simulink model "droop_model_with_current_limitation"  (R2018a)
settings: Solver=ode23tb  StartTime=0.0  StopTime=Tend  RelTol=1e-3
values from neighbouring files (symbols this model uses):
  C_4 = 0.1670*C_b    (= 1.00487241952e-06)    [VSM.m]    (also in dVOC.m; droop.m; droop_with_current_limitation.m; matching.m)
  C_6 = 0.2835*C_b    (= 1.70587623314e-06)    [VSM.m]    (also in dVOC.m; droop.m; droop_with_current_limitation.m; matching.m)
  C_8 = 0.2275*C_b    (= 1.36891302659e-06)    [VSM.m]    (also in dVOC.m; droop.m; droop_with_current_limitation.m; matching.m)
  C_dc = 0.008*(n)    (= 1.6)    [VSM.m]    (also in dVOC.m; droop.m; droop_with_current_limitation.m; matching.m)
  C_f = n*300*10^-6    (= 0.06)    [VSM.m]    (also in dVOC.m; droop.m; droop_with_current_limitation.m; matching.m)
  droop_percentage = 1    [VSM.m]    (also in dVOC.m; droop.m; droop_with_current_limitation.m; matching.m)
  I_b_LV = S_b/(sqrt(3)*V1_rms)    [VSM.m]    (also in dVOC.m; droop.m; droop_with_current_limitation.m = sqrt(2)*S_b/(sqrt(3)*V1_rms); matching.m)
  i_ll = -1.15*(S_b/Vdc_n)-i_loss_dc    [VSM.m]    (also in dVOC.m; droop.m; droop_with_current_limitation.m; matching.m)
  i_ul = 1.15*(S_b/Vdc_n)+i_loss_dc    [VSM.m]    (also in dVOC.m; droop.m; droop_with_current_limitation.m; matching.m)
  idppu = 0.9    [droop_with_current_limitation.m]
  isatpu = 1.2    [droop_with_current_limitation.m]
  k_dc = eta_1/(Vdc_n*m_p)    [VSM.m]    (also in dVOC.m; droop.m; droop_with_current_limitation.m; matching.m)
  K_dP = 2.3*S_b    (= 230000000)    [droop_with_current_limitation.m]
  K_p = (1/Vdc_n)    [VSM.m]    (also in dVOC.m; droop.m; droop_with_current_limitation.m; matching.m)
  K_r = 1/R_dc    [VSM.m]    (also in dVOC.m; droop.m; droop_with_current_limitation.m; matching.m)
  Kff_i = 1    [VSM.m]    (also in dVOC.m; droop.m; droop_with_current_limitation.m; matching.m)
  Kff_v = 1    [VSM.m]    (also in dVOC.m; droop.m; droop_with_current_limitation.m; matching.m)
  Ki_i = (1/n)*1.19    (= 0.00595)    [VSM.m]    (also in dVOC.m; droop.m; droop_with_current_limitation.m; matching.m)
  Ki_v = (n)*1.161022    (= 232.2044)    [VSM.m]    (also in dVOC.m; droop.m; droop_with_current_limitation.m; matching.m)
  ki_v_ac = 4*5.2500e-04    (= 0.0021)    [VSM.m]    (also in dVOC.m = 0.5; droop.m = 0.5; droop_with_current_limitation.m = 0.5; matching.m = 0.5)
  Kp_i = 0.738891    [VSM.m]    (also in dVOC.m; droop.m; droop_with_current_limitation.m; matching.m)
  Kp_v = 0.52    [VSM.m]    (also in dVOC.m; droop.m; droop_with_current_limitation.m; matching.m)
  kp_v_ac = 0.001    [VSM.m]    (also in dVOC.m; droop.m; droop_with_current_limitation.m; matching.m)
  L1_pu = 1*0.0186/m    (= 0.000186)    [VSM.m]    (also in dVOC.m; droop.m; droop_with_current_limitation.m; matching.m)
  L_45 = L_lines(2)    [VSM.m]    (also in dVOC.m; droop.m; droop_with_current_limitation.m; matching.m)
  L_56 = L_lines(3)    [VSM.m]    (also in dVOC.m; droop.m; droop_with_current_limitation.m; matching.m)
  L_67 = L_lines(5)    [VSM.m]    (also in dVOC.m; droop.m; droop_with_current_limitation.m; matching.m)
  L_78 = L_lines(6)    [VSM.m]    (also in dVOC.m; droop.m; droop_with_current_limitation.m; matching.m)
  L_89 = L_lines(8)    [VSM.m]    (also in dVOC.m; droop.m; droop_with_current_limitation.m; matching.m)
  L_94 = L_lines(9)    [VSM.m]    (also in dVOC.m; droop.m; droop_with_current_limitation.m; matching.m)
  L_f = (1/n)*200*10^-6    (= 1e-06)    [VSM.m]    (also in dVOC.m; droop.m; droop_with_current_limitation.m; matching.m)
  m_p = (2*pi*0.5)/(S_b)    (= 3.14159265359e-08)    [VSM.m]    (also in dVOC.m; droop.m; droop_with_current_limitation.m; matching.m)
  n = 200    [VSM.m]    (also in dVOC.m; droop.m; droop_with_current_limitation.m; matching.m)
  ps = base/3    (= 0.75)    [VSM.m]    (also in dVOC.m; droop.m; droop_with_current_limitation.m; matching.m)
  R1_pu = 1*0.00734/m    (= 7.34e-05)    [VSM.m]    (also in dVOC.m; droop.m; droop_with_current_limitation.m; matching.m)
  R_45 = R_lines(2)    [VSM.m]    (also in dVOC.m; droop.m; droop_with_current_limitation.m; matching.m)
  R_56 = R_lines(3)    [VSM.m]    (also in dVOC.m; droop.m; droop_with_current_limitation.m; matching.m)
  R_67 = R_lines(5)    [VSM.m]    (also in dVOC.m; droop.m; droop_with_current_limitation.m; matching.m)
  R_78 = R_lines(6)    [VSM.m]    (also in dVOC.m; droop.m; droop_with_current_limitation.m; matching.m)
  R_89 = R_lines(8)    [VSM.m]    (also in dVOC.m; droop.m; droop_with_current_limitation.m; matching.m)
  R_94 = R_lines(9)    [VSM.m]    (also in dVOC.m; droop.m; droop_with_current_limitation.m; matching.m)
  R_dc = (Vdc_n/(0.05*(S_b)/Vdc_n))    [VSM.m]    (also in dVOC.m; droop.m; droop_with_current_limitation.m; matching.m)
  R_f = 0.001/n    (= 5e-06)    [VSM.m]    (also in dVOC.m; droop.m; droop_with_current_limitation.m; matching.m)
  S_b = 100*(10^6)    (= 100000000)    [VSM.m]    (also in dVOC.m; droop.m; droop_with_current_limitation.m; matching.m)
  S_bt = S_b    (= 100000000)    [VSM.m]    (also in dVOC.m; droop.m; droop_with_current_limitation.m; matching.m)
  T_en = T_load-0.5    (= 24.5)    [VSM.m]    (also in dVOC.m; droop.m; droop_with_current_limitation.m; matching.m)
  T_load = 25    [VSM.m]    (also in dVOC.m; droop.m; droop_with_current_limitation.m; matching.m)
  T_loss = Tend    (= 50)    [dVOC.m]    (also in droop.m; droop_with_current_limitation.m)
  T_ms = 0.001    [dVOC.m]    (also in droop.m; droop_with_current_limitation.m)
  T_s = 1e-4    (= 0.0001)    [VSM.m]    (also in dVOC.m; droop.m; droop_with_current_limitation.m; matching.m)
  tau_dc = 0.05    [VSM.m]    (also in dVOC.m; droop.m; droop_with_current_limitation.m; matching.m)
  tau_g = 5    [VSM.m]    (also in dVOC.m; droop.m; droop_with_current_limitation.m; matching.m)
  V1_rms = 1000    [VSM.m]    (also in dVOC.m; droop.m; droop_with_current_limitation.m; matching.m)
  V2_rms = 13800    [VSM.m]    (also in dVOC.m; droop.m; droop_with_current_limitation.m; matching.m)
  V_m = sqrt(2/3)*V1_rms    [VSM.m]    (also in dVOC.m; droop.m; droop_with_current_limitation.m; matching.m)
  Vdc_n = 3*V_m    [VSM.m]    (also in dVOC.m; droop.m; droop_with_current_limitation.m; matching.m)
  w_b = 2*pi*f_b    (= 314.159265359)    [VSM.m]    (also in dVOC.m; droop.m; droop_with_current_limitation.m; matching.m)
  w_f = 2*pi*5    (= 31.4159265359)    [VSM.m]    (also in dVOC.m; droop.m; droop_with_current_limitation.m; matching.m)
undefined symbols (not defined in the file or in its folder): D1, Delta, i_dc
libraries: powerlib x88, powerlib_meascontrol x22, cstblocks x3, simulink x2, sps_avr x1
(part 2 of 2)

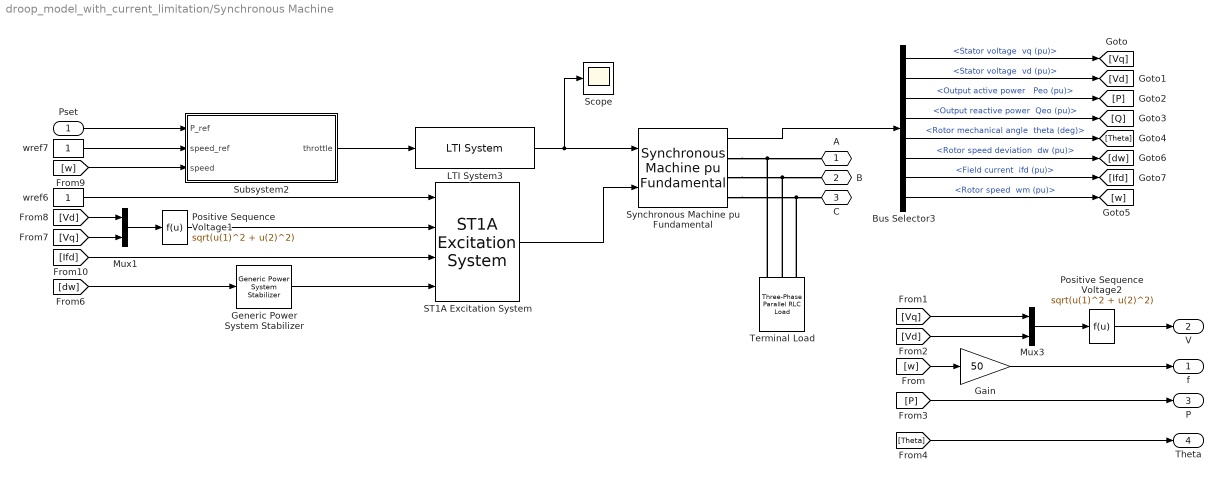
== system droop_model_with_current_limitation/Synchronous Machine ==
  Pset : Inport
  Bus Selector3 : BusSelector  OutputSignals="dq0 components.Stator voltage  vq (pu),dq0 components.Stator voltage  vd (pu),Output active power   Peo (pu),Output reactive power  Qeo (pu),Mechanical.Rotor mechanical angle  theta (deg),Mechanical.Rotor speed deviation  dw (pu),dq0 components.Field current  ifd (pu),Mechanical.Rotor speed  wm (pu)"
  Gain : Gain  Gain=50
  Generic Power System Stabilizer : powerlib/Machines/Generic Power System Stabilizer  Tsensor=30e-4  K=2.5  Twashout=2  Tleadlag1=[2*50e-3 0.1*20e-3]  Tleadlag2=[2*3 0.1*5.4]  VSlimits=2*[-0.15 0.15]  Vinit=0  Plot_On=off  MagdB_On=on  FreqRange=logspace(-2,2,500)
      settings: SourceProductName=Simscape Power Systems  SourceProductBaseCode=PS
  LTI System3 : cstblocks/LTI System  sys=ss(-1/tau_g,1/tau_g,1,[])  IC=ps
  Mux1 : Mux  Inputs=2
  Mux3 : Mux  Inputs=2
  Positive Sequence Voltage1 : Fcn  Expr=sqrt(u(1)^2 + u(2)^2)
  Positive Sequence Voltage2 : Fcn  Expr=sqrt(u(1)^2 + u(2)^2)
  ST1A Excitation System : sps_avr/ST1A Excitation System  Tr=20e-3  KaTa=[210 0.001]  VIminmax=[-999 +999]  VAminmax=[-999 999]  VRminmax=[-6.0 6.43]  KfTf=[0.001 1]  TbTc=[0 0 0 0]  KLR=1  ILR=2  Kc=0.038  v0=[1 1]  TsBlock=0
      settings: SourceProductName=Simscape Power Systems  SourceProductBaseCode=PS
  Scope : Scope
  Subsystem2 : Subsystem
  Synchronous Machine pu Fundamental : powerlib/Machines/Synchronous Machine pu Fundamental  PresetModel=No  MechanicalLoad=Mechanical power Pm  ShowDetailedParameters=on  RotorType=Salient-pole  Units=per unit fundamental parameters  MeasurementBus=off  NominalParameters="[100E6  V2_rms   50]"  Stator="[ 2.85E-03  0.114  1.19  0.36 ]"  Field="[ 5.79E-04  0.114]"  Dampers2=[0.0652, 0.5134, 0.0287, 0.2553, 7.765e-3, 0.9167 ]  Dampers1="[ 1.17E-02  0.182  1.97E-02  0.384 ]"  Mechanical=[ 3.7 0 20]  PolePairs=20  InitialConditions="[ 0  0  0  0  0  0  0  0  1 ]"  SetSaturation=off  Saturation=[0.6404,0.7127,0.8441,0.9214,0.9956,1.082,1.19,1.316,1.457;0.7,0.7698,0.8872,0.9466,0.9969,1.046,1.1,1.151,1.201]  LoadFlowParameters=[1,0,0,0,0]  TsPowergui=0  TsBlock=-1  IterativeModel=Trapezoidal non iterative  IterativeDiscreteModel=Trapezoidal non iterative  BusType=PV  Pref=0  Qref=0  Qmin=-inf  Qmax=inf  PLF=0  QLF=0
      settings: SourceProductName=Simscape Power Systems  SourceProductBaseCode=PS
  Terminal Load : powerlib/Elements/Three-Phase Parallel RLC Load  LConnTagsString=A|B|C  Configuration=Y (grounded)  NominalVoltage=V2_rms  Vabc=[1e3 1e3 1e3]  Vabcp=[1e3 1e3 1e3]  NominalFrequency=50  UnbalancedPower=off  ActivePower=1  InductivePower=0  CapacitivePower=0  Pabc=[10e3 9e3 11e3]  QLabc=[100 90 110]  QCabc=[100 90 110]  Pabcp=[10e3 9e3 11e3]  QLabcp=[100 90 110]  QCabcp=[100 90 110]  Measurements=None  LoadType=constant Z
  wref6 : Constant
  wref7 : Constant
  A : PMIOPort  Side=Right
  B : PMIOPort  Port=2  Side=Right
  C : PMIOPort  Port=3  Side=Right
  f : Outport
  V : Outport  Port=2
  P : Outport  Port=3
  Theta : Outport  Port=4
  wires:
  Gain/1 -> f/1
  Pset/1 -> Subsystem2/1(P_ref)
  Positive Sequence Voltage2/1 -> V/1
  wref7/1 -> Subsystem2/2(speed_ref)
  wref6/1 -> ST1A Excitation System/1
  Mux3/1 -> Positive Sequence Voltage2/1
  Synchronous Machine pu Fundamental/1 -> Bus Selector3/1
  [w] -> Gain/1
  [Vq] -> Mux3/1
  [Vd] -> Mux3/2
  [P] -> P/1
  [Theta] -> Theta/1
  [w] -> Subsystem2/3(speed)
  Subsystem2/1(throttle) -> LTI System3/1
  Bus Selector3/1 -> [Vq]  "<Stator voltage  vq (pu)>"
  Bus Selector3/2 -> [Vd]  "<Stator voltage  vd (pu)>"
  Bus Selector3/3 -> [P]  "<Output active power   Peo (pu)>"
  Bus Selector3/4 -> [Q]  "<Output reactive power  Qeo (pu)>"
  Bus Selector3/5 -> [Theta]  "<Rotor mechanical angle  theta (deg)>"
  Bus Selector3/6 -> [dw]  "<Rotor speed deviation  dw (pu)>"
  Bus Selector3/7 -> [Ifd]  "<Field current  ifd (pu)>"
  Bus Selector3/8 -> [w]  "<Rotor speed  wm (pu)>"
  LTI System3/1 -> Scope/1, Synchronous Machine pu Fundamental/1
  Generic Power System Stabilizer/1 -> ST1A Excitation System/4
  [dw] -> Generic Power System Stabilizer/1
  [Ifd] -> ST1A Excitation System/3
  Mux1/1 -> Positive Sequence Voltage1/1
  [Vd] -> Mux1/1
  [Vq] -> Mux1/2
  Positive Sequence Voltage1/1 -> ST1A Excitation System/2
  ST1A Excitation System/1 -> Synchronous Machine pu Fundamental/2
  connections:
  Terminal Load/LConn1 -- Synchronous Machine pu Fundamental/RConn1 -- A/RConn1
  Terminal Load/LConn3 -- Synchronous Machine pu Fundamental/RConn3 -- C/RConn1
  Terminal Load/LConn2 -- Synchronous Machine pu Fundamental/RConn2 -- B/RConn1

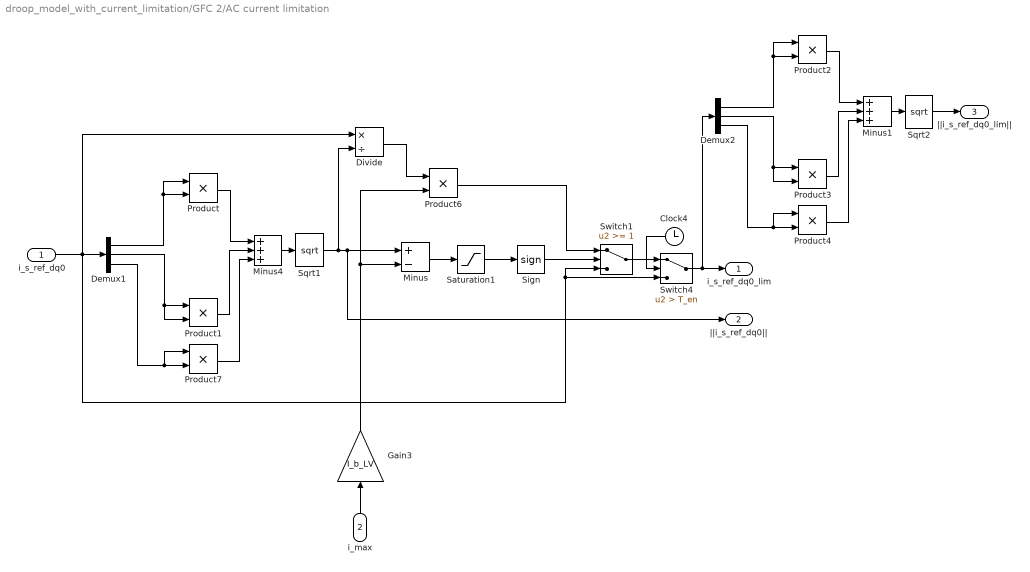
== system droop_model_with_current_limitation/GFC 2/AC current limitation ==
  i_s_ref_dq0 : Inport
  i_max : Inport  Port=2
  Clock4 : Clock
  Demux1 : Demux  Outputs=3
  Demux2 : Demux  Outputs=3
  Divide : Product  Inputs=*/
  Gain3 : Gain  Gain=I_b_LV
  Minus : Sum  Inputs=+-
  Minus1 : Sum  Inputs=+++
  Minus4 : Sum  Inputs=+++
  Product{,1..4,6..7} (7 alike) : Product  RndMeth=Zero
  Saturation1 : Saturate  UpperLimit=inf  LowerLimit=0
  Sign : Signum
  Sqrt1 : Sqrt  SaturateOnIntegerOverflow=on
  Sqrt2 : Sqrt  SaturateOnIntegerOverflow=on
  Switch1 : Switch  Threshold=1
  Switch4 : Switch  Criteria=u2 > Threshold  Threshold=T_en
  i_s_ref_dq0_lim : Outport
  ||i_s_ref_dq0|| : Outport  Port=2
  ||i_s_ref_dq0_lim|| : Outport  Port=3
  wires:
  i_max/1 -> Gain3/1
  Minus/1 -> Saturation1/1
  Sqrt1/1 -> Divide/2, ||i_s_ref_dq0||/1, Minus/1
  Minus4/1 -> Sqrt1/1
  Demux1/1 -> Product/2, Product/1
  Product1/1 -> Minus4/2
  Product/1 -> Minus4/1
  Demux1/2 -> Product1/1, Product1/2
  Saturation1/1 -> Sign/1
  Sign/1 -> Switch1/2
  Divide/1 -> Product6/1
  Product6/1 -> Switch1/1
  Product7/1 -> Minus4/3
  Demux1/3 -> Product7/1, Product7/2
  Switch4/1 -> Demux2/1, i_s_ref_dq0_lim/1
  i_s_ref_dq0/1 -> Divide/1, Demux1/1, Switch4/3, Switch1/3
  Clock4/1 -> Switch4/2
  Switch1/1 -> Switch4/1
  Gain3/1 -> Minus/2, Product6/2
  Product2/1 -> Minus1/1
  Demux2/3 -> Product4/1, Product4/2
  Product4/1 -> Minus1/3
  Demux2/1 -> Product2/2, Product2/1
  Product3/1 -> Minus1/2
  Demux2/2 -> Product3/1, Product3/2
  Minus1/1 -> Sqrt2/1
  Sqrt2/1 -> ||i_s_ref_dq0_lim||/1

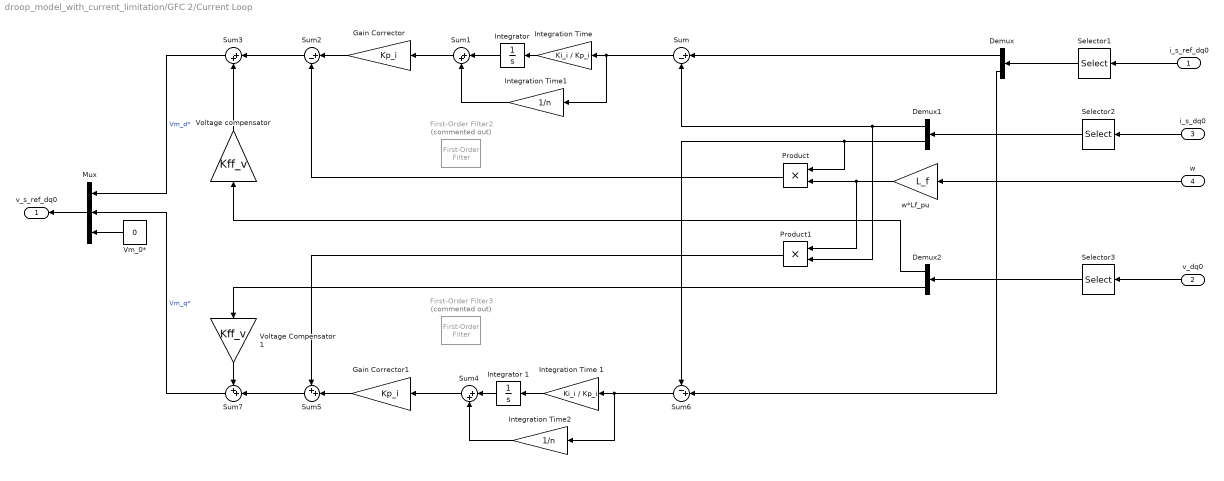
== system droop_model_with_current_limitation/GFC 2/Current Loop ==
  i_s_ref_dq0 : Inport
  v_dq0 : Inport  Port=2
  i_s_dq0 : Inport  Port=3
  w : Inport  Port=4
  Demux : Demux  Outputs=2
  Demux1 : Demux  Outputs=2
  Demux2 : Demux  Outputs=2
  First-Order Filter2 : powerlib_meascontrol/Filters/First-Order Filter  Commented=on  FilterType=Lowpass  Tc=25e-3  Ts=0  Initialize=on  Vac_Init=[0, 0, 50]  Vdc_Init=1  PlotResponse=off  FreqRange="[0,  200,  1]"
      settings: SourceProductName=Simscape Power Systems
  First-Order Filter3 : powerlib_meascontrol/Filters/First-Order Filter  Commented=on  FilterType=Lowpass  Tc=25e-3  Ts=0  Initialize=on  Vac_Init=[0, 0, 50]  Vdc_Init=0  PlotResponse=off  FreqRange="[0,  200,  1]"
      settings: SourceProductName=Simscape Power Systems
  Gain Corrector : Gain  Gain=Kp_i
  Gain Corrector1 : Gain  Gain=Kp_i
  Integration Time : Gain  Gain=Ki_i / Kp_i
  Integration Time 1 : Gain  Gain=Ki_i / Kp_i
  Integration Time1 : Gain  Gain=1/n
  Integration Time2 : Gain  Gain=1/n
  Integrator : Integrator  InitialCondition=0.0001
  Integrator 1 : Integrator
  Mux : Mux  Inputs=3
  Product : Product  RndMeth=Zero
  Product1 : Product  RndMeth=Zero
  Selector1 : Selector  InputPortWidth=3  IndexOptions=Index vector (dialog)  Indices=[1 2]  OutputSizes=1
  Selector2 : Selector  InputPortWidth=3  IndexOptions=Index vector (dialog)  Indices=[1 2]  OutputSizes=1
  Selector3 : Selector  InputPortWidth=3  IndexOptions=Index vector (dialog)  Indices=[1 2]  OutputSizes=1
  Sum : Sum  Inputs=|+-
  Sum1 : Sum  Inputs=|++
  Sum2 : Sum  Inputs=|+-
  Sum3 : Sum  Inputs=|++
  Sum4 : Sum  Inputs=|++
  Sum5 : Sum  Inputs=++|
  Sum6 : Sum  Inputs=-+|
  Sum7 : Sum  Inputs=++|
  Vm_0* : Constant  Value=0
  Voltage Compensator 1 : Gain  Gain=Kff_v
  Voltage compensator : Gain  Gain=Kff_v
  w*Lf_pu : Gain  Gain=L_f
  v_s_ref_dq0 : Outport
  wires:
  Sum/1 -> Integration Time/1, Integration Time1/1
  Integration Time 1/1 -> Integrator 1/1
  Integration Time/1 -> Integrator/1
  Sum5/1 -> Sum7/2
  Sum6/1 -> Integration Time 1/1, Integration Time2/1
  Demux/1 -> Sum/1
  Sum3/1 -> Mux/1  "Vm_d*"
  Sum7/1 -> Mux/2  "Vm_q*"
  Demux2/2 -> Voltage Compensator 1/1
  Voltage Compensator 1/1 -> Sum7/1
  Product/1 -> Sum2/2
  w*Lf_pu/1 -> Product1/1, Product/2
  i_s_ref_dq0/1 -> Selector1/1
  v_dq0/1 -> Selector3/1
  Integrator 1/1 -> Sum4/1
  Voltage compensator/1 -> Sum3/2
  Sum1/1 -> Gain Corrector/1
  Sum2/1 -> Sum3/1
  Sum4/1 -> Gain Corrector1/1
  Demux/2 -> Sum6/2
  Selector1/1 -> Demux/1
  Gain Corrector/1 -> Sum2/1
  w/1 -> w*Lf_pu/1
  Mux/1 -> v_s_ref_dq0/1
  Selector2/1 -> Demux1/1
  i_s_dq0/1 -> Selector2/1
  Selector3/1 -> Demux2/1
  Demux1/2 -> Product/1, Sum6/1
  Vm_0*/1 -> Mux/3
  Integrator/1 -> Sum1/1
  Demux1/1 -> Product1/2, Sum/2
  Demux2/1 -> Voltage compensator/1
  Product1/1 -> Sum5/1
  Gain Corrector1/1 -> Sum5/2
  Integration Time1/1 -> Sum1/2
  Integration Time2/1 -> Sum4/2

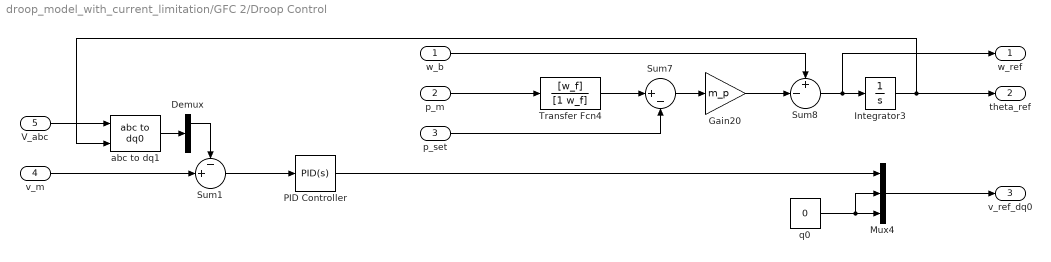
== system droop_model_with_current_limitation/GFC 2/Droop Control ==
  w_b : Inport
  p_m : Inport  Port=2
  p_set : Inport  Port=3
  v_m : Inport  Port=4
  V_abc : Inport  Port=5
  Demux : Demux  Outputs=3
  Gain20 : Gain  Gain=m_p
  Integrator3 : Integrator
  Mux4 : Mux  Inputs=3
  PID Controller : simulink/Continuous/PID Controller  Controller=PID  TimeDomain=Continuous-time  SampleTime=-1  IntegratorMethod=Forward Euler  FilterMethod=Forward Euler  Form=Parallel  UseFilter=on  ControllerParametersSource=internal  P=kp_v_ac  I=ki_v_ac  D=0  N=100  InitialConditionSource=internal  InitialConditionForIntegrator=0  InitialConditionForFilter=0  ExternalReset=none  LimitOutput=off  UpperSaturationLimit=inf  LowerSaturationLimit=-inf  LinearizeAsGain=on  AntiWindupMode=back-calculation  Kb=1  TrackingMode=off  Kt=1  PParamMin=[]  PParamMax=[]  IParamMin=[]  IParamMax=[]  DParamMin=[]  DParamMax=[]  NParamMin=[]  NParamMax=[]  KbParamMin=[]  KbParamMax=[]  KtParamMin=[]  KtParamMax=[]  POutMin=[]  POutMax=[]  IOutMin=[]  IOutMax=[]  DOutMin=[]  DOutMax=[]  NOutMin=[]  NOutMax=[]  KbOutMin=[]  KbOutMax=[]  KtOutMin=[]  KtOutMax=[]  IntegratorOutMin=[]  IntegratorOutMax=[]  FilterOutMin=[]  FilterOutMax=[]  SumOutMin=[]  SumOutMax=[]  SumI1OutMin=[]  SumI1OutMax=[]  SumI2OutMin=[]  SumI2OutMax=[]  SumI3OutMin=[]  SumI3OutMax=[]  SumDOutMin=[]  SumDOutMax=[]  SaturationOutMin=[]  SaturationOutMax=[]  IntegratorContinuousStateAttributes=''  IntegratorStateMustResolveToSignalObject=off  IntegratorRTWStateStorageClass=Auto  FilterContinuousStateAttributes=''  FilterStateMustResolveToSignalObject=off  FilterRTWStateStorageClass=Auto  DifferentiatorICPrevScaledInput=0  DifferentiatorOutMin=[]  DifferentiatorOutMax=[]  InitialConditionSetting=State (most efficient)  FilterDiffOutCoefMin=[]  FilterDiffOutCoefMax=[]  SumDenOutMin=[]  SumDenOutMax=[]  SumNumOutMin=[]  SumNumOutMax=[]  ReciprocalOutMin=[]  ReciprocalOutMax=[]  DivideOutMin=[]  DivideOutMax=[]  TunerSelectOption=Transfer Function Based (PID Tuner App)
  Sum1 : Sum  Inputs=-+|
  Sum7 : Sum  Inputs=|+-
  Sum8 : Sum  Inputs=+-|
  Transfer Fcn4 : TransferFcn  Numerator=[w_f]  Denominator=[1 w_f]
  abc to dq1 : powerlib_meascontrol/Transformations/abc to dq0  Alignment=90 degrees behind phase A axis
  q0 : Constant  Value=0
  w_ref : Outport
  theta_ref : Outport  Port=2
  v_ref_dq0 : Outport  Port=3
  wires:
  Demux/1 -> Sum1/1
  abc to dq1/1 -> Demux/1
  Transfer Fcn4/1 -> Sum7/1
  Mux4/1 -> v_ref_dq0/1
  q0/1 -> Mux4/3, Mux4/2
  Sum8/1 -> Integrator3/1, w_ref/1
  Gain20/1 -> Sum8/2
  Sum7/1 -> Gain20/1
  p_m/1 -> Transfer Fcn4/1
  p_set/1 -> Sum7/2
  w_b/1 -> Sum8/1
  V_abc/1 -> abc to dq1/1
  Sum1/1 -> PID Controller/1
  Integrator3/1 -> abc to dq1/2, theta_ref/1
  v_m/1 -> Sum1/2
  PID Controller/1 -> Mux4/1

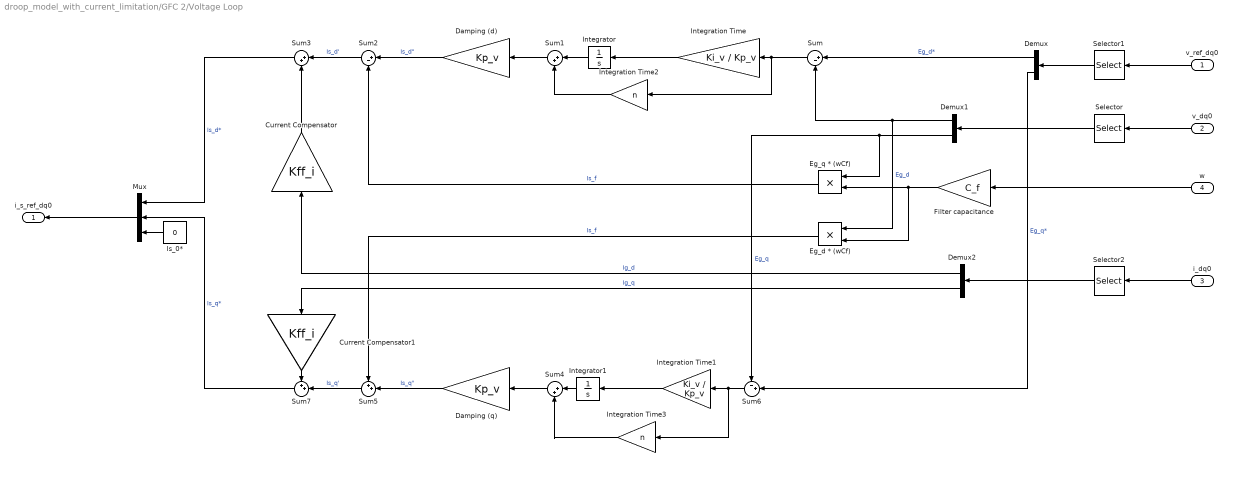
== system droop_model_with_current_limitation/GFC 2/Voltage Loop ==
  v_ref_dq0 : Inport
  v_dq0 : Inport  Port=2
  i_dq0 : Inport  Port=3
  w : Inport  Port=4
  Current Compensator : Gain  Gain=Kff_i
  Current Compensator1 : Gain  Gain=Kff_i
  Damping (d) : Gain  Gain=Kp_v
  Damping (q) : Gain  Gain=Kp_v
  Demux : Demux  Outputs=2
  Demux1 : Demux  Outputs=2
  Demux2 : Demux  Outputs=2
  Eg_d * (wCf) : Product  RndMeth=Zero
  "Eg_q * (wCf) " : Product  RndMeth=Zero
  Filter capacitance : Gain  Gain=C_f
  Integration Time : Gain  Gain=Ki_v / Kp_v
  Integration Time1 : Gain  Gain=Ki_v / Kp_v
  Integration Time2 : Gain  Gain=n
  Integration Time3 : Gain  Gain=n
  Integrator : Integrator
  Integrator1 : Integrator
  Is_0* : Constant  Value=0
  Mux : Mux  Inputs=3
  Selector : Selector  InputPortWidth=3  IndexOptions=Index vector (dialog)  Indices=[1 2]  OutputSizes=1
  Selector1 : Selector  InputPortWidth=3  IndexOptions=Index vector (dialog)  Indices=[1 2]  OutputSizes=1
  Selector2 : Selector  InputPortWidth=3  IndexOptions=Index vector (dialog)  Indices=[1 2]  OutputSizes=1
  Sum : Sum  Inputs=|+-
  Sum1 : Sum  Inputs=|++
  Sum2 : Sum  Inputs=|+-
  Sum3 : Sum  Inputs=|++
  Sum4 : Sum  Inputs=|++
  Sum5 : Sum  Inputs=++|
  Sum6 : Sum  Inputs=-+|
  Sum7 : Sum  Inputs=++|
  i_s_ref_dq0 : Outport
  wires:
  Is_0*/1 -> Mux/3
  w/1 -> Filter capacitance/1
  Integrator1/1 -> Sum4/1
  Demux/2 -> Sum6/2  "Eg_q*"
  v_ref_dq0/1 -> Selector1/1
  Eg_d * (wCf)/1 -> Sum5/1  "Is_f"
  Sum7/1 -> Mux/2  "Is_q*"
  Demux2/2 -> Current Compensator1/1  "Ig_q"
  Demux/1 -> Sum/1  "Eg_d*"
  Sum6/1 -> Integration Time3/1, Integration Time1/1
  Demux2/1 -> Current Compensator/1  "Ig_d"
  Sum2/1 -> Sum3/1  "Is_d'"
  Current Compensator/1 -> Sum3/2
  Demux1/1 -> Eg_d * (wCf)/1, Sum/2  "Eg_d"
  Current Compensator1/1 -> Sum7/1
  "Eg_q * (wCf) "/1 -> Sum2/2  "Is_f"
  Demux1/2 -> "Eg_q * (wCf) "/1, Sum6/1  "Eg_q"
  Filter capacitance/1 -> "Eg_q * (wCf) "/2, Eg_d * (wCf)/2
  Damping (d)/1 -> Sum2/1  "Is_d\""
  i_dq0/1 -> Selector2/1
  Sum5/1 -> Sum7/2  "Is_q'"
  Sum1/1 -> Damping (d)/1
  Integrator/1 -> Sum1/1
  Sum4/1 -> Damping (q)/1
  Sum3/1 -> Mux/1  "Is_d*"
  v_dq0/1 -> Selector/1
  Damping (q)/1 -> Sum5/2  "Is_q\""
  Selector/1 -> Demux1/1
  Selector1/1 -> Demux/1
  Selector2/1 -> Demux2/1
  Mux/1 -> i_s_ref_dq0/1
  Sum/1 -> Integration Time/1, Integration Time2/1
  Integration Time2/1 -> Sum1/2
  Integration Time3/1 -> Sum4/2
  Integration Time/1 -> Integrator/1
  Integration Time1/1 -> Integrator1/1

== system droop_model_with_current_limitation/GFC 2/power set-point modification ==
  i_s_dq0 : Inport
  i_thr : Inport  Port=2
  Dot Product : DotProduct  InputSameDT=on  OutDataTypeStr=Inherit: Inherit via internal rule
  Gain : Gain  Gain=[eye(2),zeros(2,1)]  Multiplication=Matrix(K*u) (u vector)
  Gain1 : Gain  Gain=K_dP/I_b_LV
  Gain2 : Gain  Gain=I_b_LV
  Saturation : Saturate  UpperLimit=inf  LowerLimit=0
  Sqrt : Sqrt  SaturateOnIntegerOverflow=on
  Sum : Sum  Inputs=|+-
  delta P* : Outport
  wires:
  i_s_dq0/1 -> Gain/1
  Dot Product/1 -> Sqrt/1
  Gain/1 -> Dot Product/1, Dot Product/2
  Sqrt/1 -> Sum/1
  i_thr/1 -> Gain2/1
  Sum/1 -> Saturation/1
  Gain1/1 -> delta P*/1
  Saturation/1 -> Gain1/1
  Gain2/1 -> Sum/2

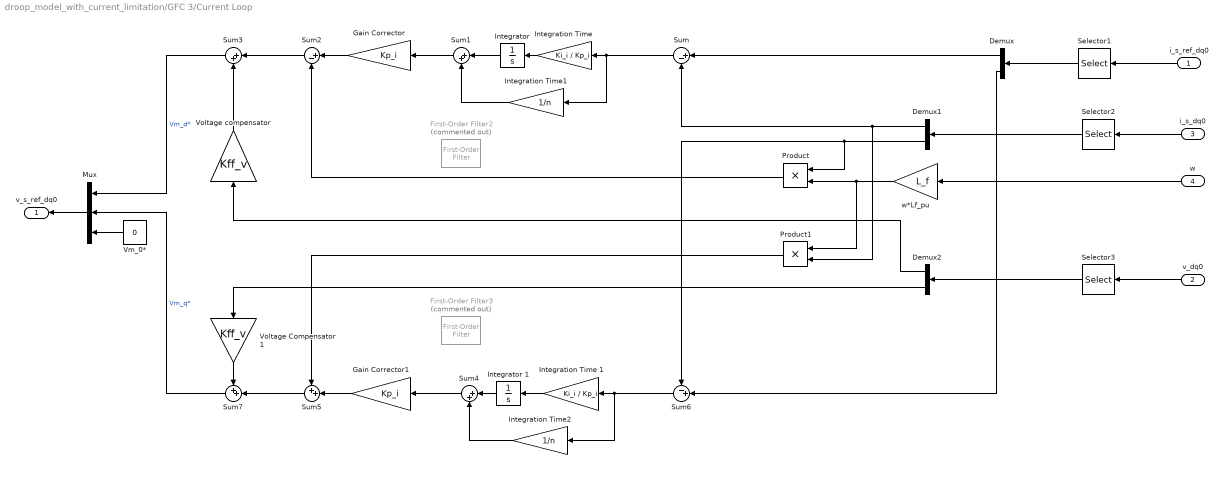
== system droop_model_with_current_limitation/GFC 3/Current Loop ==
  i_s_ref_dq0 : Inport
  v_dq0 : Inport  Port=2
  i_s_dq0 : Inport  Port=3
  w : Inport  Port=4
  Demux : Demux  Outputs=2
  Demux1 : Demux  Outputs=2
  Demux2 : Demux  Outputs=2
  First-Order Filter2 : powerlib_meascontrol/Filters/First-Order Filter  Commented=on  FilterType=Lowpass  Tc=25e-3  Ts=0  Initialize=on  Vac_Init=[0, 0, 50]  Vdc_Init=1  PlotResponse=off  FreqRange="[0,  200,  1]"
      settings: SourceProductName=Simscape Power Systems
  First-Order Filter3 : powerlib_meascontrol/Filters/First-Order Filter  Commented=on  FilterType=Lowpass  Tc=25e-3  Ts=0  Initialize=on  Vac_Init=[0, 0, 50]  Vdc_Init=0  PlotResponse=off  FreqRange="[0,  200,  1]"
      settings: SourceProductName=Simscape Power Systems
  Gain Corrector : Gain  Gain=Kp_i
  Gain Corrector1 : Gain  Gain=Kp_i
  Integration Time : Gain  Gain=Ki_i / Kp_i
  Integration Time 1 : Gain  Gain=Ki_i / Kp_i
  Integration Time1 : Gain  Gain=1/n
  Integration Time2 : Gain  Gain=1/n
  Integrator : Integrator  InitialCondition=0.0001
  Integrator 1 : Integrator
  Mux : Mux  Inputs=3
  Product : Product  RndMeth=Zero
  Product1 : Product  RndMeth=Zero
  Selector1 : Selector  InputPortWidth=3  IndexOptions=Index vector (dialog)  Indices=[1 2]  OutputSizes=1
  Selector2 : Selector  InputPortWidth=3  IndexOptions=Index vector (dialog)  Indices=[1 2]  OutputSizes=1
  Selector3 : Selector  InputPortWidth=3  IndexOptions=Index vector (dialog)  Indices=[1 2]  OutputSizes=1
  Sum : Sum  Inputs=|+-
  Sum1 : Sum  Inputs=|++
  Sum2 : Sum  Inputs=|+-
  Sum3 : Sum  Inputs=|++
  Sum4 : Sum  Inputs=|++
  Sum5 : Sum  Inputs=++|
  Sum6 : Sum  Inputs=-+|
  Sum7 : Sum  Inputs=++|
  Vm_0* : Constant  Value=0
  Voltage Compensator 1 : Gain  Gain=Kff_v
  Voltage compensator : Gain  Gain=Kff_v
  w*Lf_pu : Gain  Gain=L_f
  v_s_ref_dq0 : Outport
  wires:
  Integration Time2/1 -> Sum4/2
  Integration Time1/1 -> Sum1/2
  Gain Corrector1/1 -> Sum5/2
  Product1/1 -> Sum5/1
  Demux2/1 -> Voltage compensator/1
  Demux1/1 -> Sum/2, Product1/2
  Integrator/1 -> Sum1/1
  Vm_0*/1 -> Mux/3
  Demux1/2 -> Sum6/1, Product/1
  Selector3/1 -> Demux2/1
  i_s_dq0/1 -> Selector2/1
  Selector2/1 -> Demux1/1
  Mux/1 -> v_s_ref_dq0/1
  w/1 -> w*Lf_pu/1
  Gain Corrector/1 -> Sum2/1
  Selector1/1 -> Demux/1
  Demux/2 -> Sum6/2
  Sum4/1 -> Gain Corrector1/1
  Sum2/1 -> Sum3/1
  Sum1/1 -> Gain Corrector/1
  Voltage compensator/1 -> Sum3/2
  Integrator 1/1 -> Sum4/1
  v_dq0/1 -> Selector3/1
  i_s_ref_dq0/1 -> Selector1/1
  w*Lf_pu/1 -> Product/2, Product1/1
  Product/1 -> Sum2/2
  Voltage Compensator 1/1 -> Sum7/1
  Demux2/2 -> Voltage Compensator 1/1
  Sum7/1 -> Mux/2  "Vm_q*"
  Sum3/1 -> Mux/1  "Vm_d*"
  Demux/1 -> Sum/1
  Sum6/1 -> Integration Time2/1, Integration Time 1/1
  Sum5/1 -> Sum7/2
  Integration Time/1 -> Integrator/1
  Integration Time 1/1 -> Integrator 1/1
  Sum/1 -> Integration Time1/1, Integration Time/1

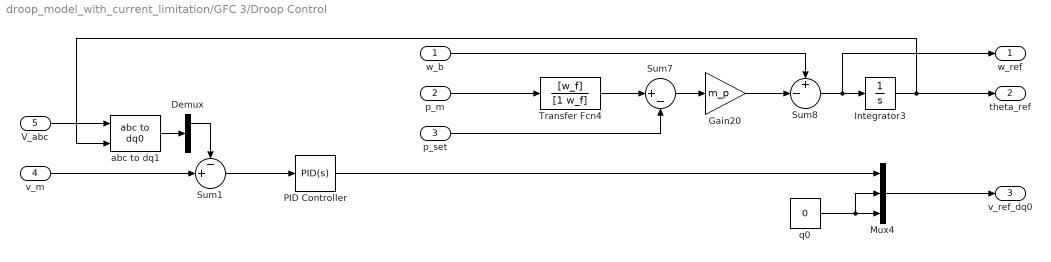
== system droop_model_with_current_limitation/GFC 3/Droop Control ==
  w_b : Inport
  p_m : Inport  Port=2
  p_set : Inport  Port=3
  v_m : Inport  Port=4
  V_abc : Inport  Port=5
  Demux : Demux  Outputs=3
  Gain20 : Gain  Gain=m_p
  Integrator3 : Integrator
  Mux4 : Mux  Inputs=3
  PID Controller : simulink/Continuous/PID Controller  Controller=PID  TimeDomain=Continuous-time  SampleTime=-1  IntegratorMethod=Forward Euler  FilterMethod=Forward Euler  Form=Parallel  UseFilter=on  ControllerParametersSource=internal  P=kp_v_ac  I=ki_v_ac  D=0  N=100  InitialConditionSource=internal  InitialConditionForIntegrator=0  InitialConditionForFilter=0  ExternalReset=none  LimitOutput=off  UpperSaturationLimit=inf  LowerSaturationLimit=-inf  LinearizeAsGain=on  AntiWindupMode=back-calculation  Kb=1  TrackingMode=off  Kt=1  PParamMin=[]  PParamMax=[]  IParamMin=[]  IParamMax=[]  DParamMin=[]  DParamMax=[]  NParamMin=[]  NParamMax=[]  KbParamMin=[]  KbParamMax=[]  KtParamMin=[]  KtParamMax=[]  POutMin=[]  POutMax=[]  IOutMin=[]  IOutMax=[]  DOutMin=[]  DOutMax=[]  NOutMin=[]  NOutMax=[]  KbOutMin=[]  KbOutMax=[]  KtOutMin=[]  KtOutMax=[]  IntegratorOutMin=[]  IntegratorOutMax=[]  FilterOutMin=[]  FilterOutMax=[]  SumOutMin=[]  SumOutMax=[]  SumI1OutMin=[]  SumI1OutMax=[]  SumI2OutMin=[]  SumI2OutMax=[]  SumI3OutMin=[]  SumI3OutMax=[]  SumDOutMin=[]  SumDOutMax=[]  SaturationOutMin=[]  SaturationOutMax=[]  IntegratorContinuousStateAttributes=''  IntegratorStateMustResolveToSignalObject=off  IntegratorRTWStateStorageClass=Auto  FilterContinuousStateAttributes=''  FilterStateMustResolveToSignalObject=off  FilterRTWStateStorageClass=Auto  DifferentiatorICPrevScaledInput=0  DifferentiatorOutMin=[]  DifferentiatorOutMax=[]  InitialConditionSetting=State (most efficient)  FilterDiffOutCoefMin=[]  FilterDiffOutCoefMax=[]  SumDenOutMin=[]  SumDenOutMax=[]  SumNumOutMin=[]  SumNumOutMax=[]  ReciprocalOutMin=[]  ReciprocalOutMax=[]  DivideOutMin=[]  DivideOutMax=[]  TunerSelectOption=Transfer Function Based (PID Tuner App)
  Sum1 : Sum  Inputs=-+|
  Sum7 : Sum  Inputs=|+-
  Sum8 : Sum  Inputs=+-|
  Transfer Fcn4 : TransferFcn  Numerator=[w_f]  Denominator=[1 w_f]
  abc to dq1 : powerlib_meascontrol/Transformations/abc to dq0  Alignment=90 degrees behind phase A axis
  q0 : Constant  Value=0
  w_ref : Outport
  theta_ref : Outport  Port=2
  v_ref_dq0 : Outport  Port=3
  wires:
  PID Controller/1 -> Mux4/1
  v_m/1 -> Sum1/2
  Integrator3/1 -> theta_ref/1, abc to dq1/2
  Sum1/1 -> PID Controller/1
  V_abc/1 -> abc to dq1/1
  w_b/1 -> Sum8/1
  p_set/1 -> Sum7/2
  p_m/1 -> Transfer Fcn4/1
  Sum7/1 -> Gain20/1
  Gain20/1 -> Sum8/2
  Sum8/1 -> w_ref/1, Integrator3/1
  q0/1 -> Mux4/2, Mux4/3
  Mux4/1 -> v_ref_dq0/1
  Transfer Fcn4/1 -> Sum7/1
  abc to dq1/1 -> Demux/1
  Demux/1 -> Sum1/1

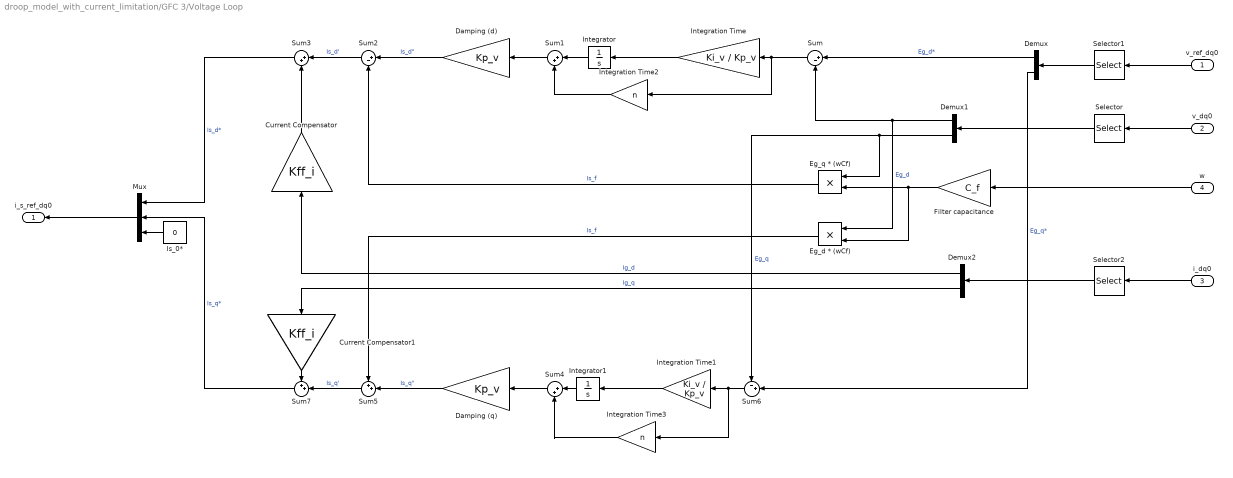
== system droop_model_with_current_limitation/GFC 3/Voltage Loop ==
  v_ref_dq0 : Inport
  v_dq0 : Inport  Port=2
  i_dq0 : Inport  Port=3
  w : Inport  Port=4
  Current Compensator : Gain  Gain=Kff_i
  Current Compensator1 : Gain  Gain=Kff_i
  Damping (d) : Gain  Gain=Kp_v
  Damping (q) : Gain  Gain=Kp_v
  Demux : Demux  Outputs=2
  Demux1 : Demux  Outputs=2
  Demux2 : Demux  Outputs=2
  Eg_d * (wCf) : Product  RndMeth=Zero
  "Eg_q * (wCf) " : Product  RndMeth=Zero
  Filter capacitance : Gain  Gain=C_f
  Integration Time : Gain  Gain=Ki_v / Kp_v
  Integration Time1 : Gain  Gain=Ki_v / Kp_v
  Integration Time2 : Gain  Gain=n
  Integration Time3 : Gain  Gain=n
  Integrator : Integrator
  Integrator1 : Integrator
  Is_0* : Constant  Value=0
  Mux : Mux  Inputs=3
  Selector : Selector  InputPortWidth=3  IndexOptions=Index vector (dialog)  Indices=[1 2]  OutputSizes=1
  Selector1 : Selector  InputPortWidth=3  IndexOptions=Index vector (dialog)  Indices=[1 2]  OutputSizes=1
  Selector2 : Selector  InputPortWidth=3  IndexOptions=Index vector (dialog)  Indices=[1 2]  OutputSizes=1
  Sum : Sum  Inputs=|+-
  Sum1 : Sum  Inputs=|++
  Sum2 : Sum  Inputs=|+-
  Sum3 : Sum  Inputs=|++
  Sum4 : Sum  Inputs=|++
  Sum5 : Sum  Inputs=++|
  Sum6 : Sum  Inputs=-+|
  Sum7 : Sum  Inputs=++|
  i_s_ref_dq0 : Outport
  wires:
  Integration Time1/1 -> Integrator1/1
  Integration Time/1 -> Integrator/1
  Integration Time3/1 -> Sum4/2
  Integration Time2/1 -> Sum1/2
  Sum/1 -> Integration Time2/1, Integration Time/1
  Mux/1 -> i_s_ref_dq0/1
  Selector2/1 -> Demux2/1
  Selector1/1 -> Demux/1
  Selector/1 -> Demux1/1
  Damping (q)/1 -> Sum5/2  "Is_q\""
  v_dq0/1 -> Selector/1
  Sum3/1 -> Mux/1  "Is_d*"
  Sum4/1 -> Damping (q)/1
  Integrator/1 -> Sum1/1
  Sum1/1 -> Damping (d)/1
  Sum5/1 -> Sum7/2  "Is_q'"
  i_dq0/1 -> Selector2/1
  Damping (d)/1 -> Sum2/1  "Is_d\""
  Filter capacitance/1 -> Eg_d * (wCf)/2, "Eg_q * (wCf) "/2
  Demux1/2 -> Sum6/1, "Eg_q * (wCf) "/1  "Eg_q"
  "Eg_q * (wCf) "/1 -> Sum2/2  "Is_f"
  Current Compensator1/1 -> Sum7/1
  Demux1/1 -> Sum/2, Eg_d * (wCf)/1  "Eg_d"
  Current Compensator/1 -> Sum3/2
  Sum2/1 -> Sum3/1  "Is_d'"
  Demux2/1 -> Current Compensator/1  "Ig_d"
  Sum6/1 -> Integration Time1/1, Integration Time3/1
  Demux/1 -> Sum/1  "Eg_d*"
  Demux2/2 -> Current Compensator1/1  "Ig_q"
  Sum7/1 -> Mux/2  "Is_q*"
  Eg_d * (wCf)/1 -> Sum5/1  "Is_f"
  v_ref_dq0/1 -> Selector1/1
  Demux/2 -> Sum6/2  "Eg_q*"
  Integrator1/1 -> Sum4/1
  w/1 -> Filter capacitance/1
  Is_0*/1 -> Mux/3

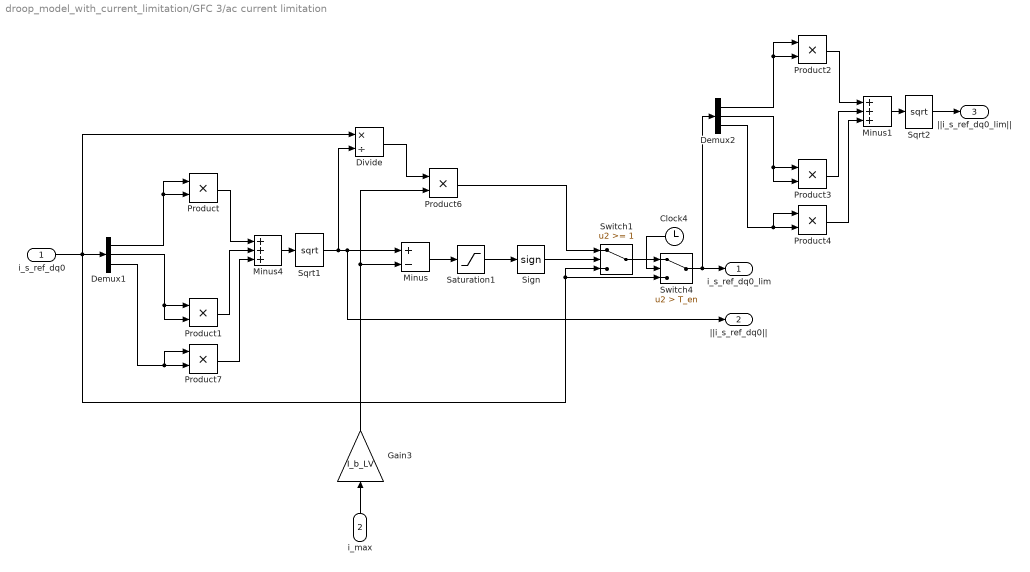
== system droop_model_with_current_limitation/GFC 3/ac current limitation ==
  i_s_ref_dq0 : Inport
  i_max : Inport  Port=2
  Clock4 : Clock
  Demux1 : Demux  Outputs=3
  Demux2 : Demux  Outputs=3
  Divide : Product  Inputs=*/
  Gain3 : Gain  Gain=I_b_LV
  Minus : Sum  Inputs=+-
  Minus1 : Sum  Inputs=+++
  Minus4 : Sum  Inputs=+++
  Product{,1..4,6..7} (7 alike) : Product  RndMeth=Zero
  Saturation1 : Saturate  UpperLimit=inf  LowerLimit=0
  Sign : Signum
  Sqrt1 : Sqrt  SaturateOnIntegerOverflow=on
  Sqrt2 : Sqrt  SaturateOnIntegerOverflow=on
  Switch1 : Switch  Threshold=1
  Switch4 : Switch  Criteria=u2 > Threshold  Threshold=T_en
  i_s_ref_dq0_lim : Outport
  ||i_s_ref_dq0|| : Outport  Port=2
  ||i_s_ref_dq0_lim|| : Outport  Port=3
  wires:
  Sqrt2/1 -> ||i_s_ref_dq0_lim||/1
  Minus1/1 -> Sqrt2/1
  Demux2/2 -> Product3/2, Product3/1
  Product3/1 -> Minus1/2
  Demux2/1 -> Product2/1, Product2/2
  Product4/1 -> Minus1/3
  Demux2/3 -> Product4/2, Product4/1
  Product2/1 -> Minus1/1
  Gain3/1 -> Product6/2, Minus/2
  Switch1/1 -> Switch4/1
  Clock4/1 -> Switch4/2
  i_s_ref_dq0/1 -> Switch1/3, Switch4/3, Demux1/1, Divide/1
  Switch4/1 -> i_s_ref_dq0_lim/1, Demux2/1
  Demux1/3 -> Product7/2, Product7/1
  Product7/1 -> Minus4/3
  Product6/1 -> Switch1/1
  Divide/1 -> Product6/1
  Sign/1 -> Switch1/2
  Saturation1/1 -> Sign/1
  Demux1/2 -> Product1/2, Product1/1
  Product/1 -> Minus4/1
  Product1/1 -> Minus4/2
  Demux1/1 -> Product/1, Product/2
  Minus4/1 -> Sqrt1/1
  Sqrt1/1 -> Minus/1, ||i_s_ref_dq0||/1, Divide/2
  Minus/1 -> Saturation1/1
  i_max/1 -> Gain3/1

== system droop_model_with_current_limitation/GFC 3/power set-point modification ==
  i_s_dq0 : Inport
  i_thr : Inport  Port=2
  Dot Product : DotProduct  InputSameDT=on  OutDataTypeStr=Inherit: Inherit via internal rule
  Gain : Gain  Gain=[eye(2),zeros(2,1)]  Multiplication=Matrix(K*u) (u vector)
  Gain1 : Gain  Gain=K_dP/I_b_LV
  Gain2 : Gain  Gain=I_b_LV
  Saturation : Saturate  UpperLimit=inf  LowerLimit=0
  Sqrt : Sqrt  SaturateOnIntegerOverflow=on
  Sum : Sum  Inputs=|+-
  delta P* : Outport
  wires:
  Gain2/1 -> Sum/2
  Saturation/1 -> Gain1/1
  Gain1/1 -> delta P*/1
  Sum/1 -> Saturation/1
  i_thr/1 -> Gain2/1
  Sqrt/1 -> Sum/1
  Gain/1 -> Dot Product/2, Dot Product/1
  Dot Product/1 -> Sqrt/1
  i_s_dq0/1 -> Gain/1

== system droop_model_with_current_limitation/Synchronous Machine/Subsystem2 ==
  P_ref : Inport
  speed_ref : Inport  Port=2
  speed : Inport  Port=3
  1/droop : Gain  Gain=1/((droop_percentage/100))
  Delta load setpoint : Sum  Inputs=+-|
  Delta speed : Sum  Inputs=-+|
  throttle : Outport
  wires:
  speed/1 -> Delta speed/2
  1/droop/1 -> Delta load setpoint/2
  Delta speed/1 -> 1/droop/1
  speed_ref/1 -> Delta speed/1
  P_ref/1 -> Delta load setpoint/1
  Delta load setpoint/1 -> throttle/1
